simulink library "icc_lib_avg_path1_n1"  (R2018b)
settings: Solver=VariableStepAuto  StartTime=0.0  StopTime=10.0  RelTol=1e-3
undefined symbols (not defined in the file or in its folder): icc_lib_avg_path, path1
libraries: simulink x34, simulink_extras x8, $bdroot x2
(part 4 of 4)

== stateflow chart icc_lib_avg_path1_n1/ICC7_egm/Chart ==
  state block
    en:
    q=4
  state wait
    entry:
    du:
    t2=temporalCount (sec);
  state q0
    en:
    q=0
  state q1
    en:
    q=1
    Sense=1
    exit:
    Sense=0
  state q3
    en:
    q=3
  state q2
    en:
    q=2
  wait -> (junction 82) : [t2>=19.999]{q=0;th=0;vreset=-67.6336;reset}
  (junction 82) -> block [order 2] : [b==1]
  (junction 82) -> q0 [order 1] : [b==0]
  (default) -> wait : {t2=0;}
  q0 -> block [order 3] : [b==1]
  block -> q0 : [b==0]
  q0 -> q1 [order 1] : [v<VT]/{vreset=v; th=0; Vmax=Vm;d2=d2i; reset}
  q0 -> q1 [order 2] : [gv>VF&&v>VT]{ vreset=v; th=v-VT/VF-VT; Vmax=func1(th,Vm);d2=func2(th,d2i);reset}
  q3 -> q0 : [v<VF]{vreset=v; reset}
  q1 -> q2 : [ v >Vmax ]{vreset=v; reset}
  q2 -> q3 : [v<VR]{vreset=v; reset}
  data: vmax function_output double; theta function_input; vm function_input; d2out function_output double; theta function_input; d2in function_input; v input double; q output; vreset output; gv input double; Vmm input; VT input; Vm input; VR input; VF input; th local; Vmax local; t2 local; d2i input; d2 output; b input; Sense output
  events: reset output EITHER_EDGE_EVENT
  function vmax = func1(theta,vm):
    | function vmax = func1(theta,vm)
    | 
    | m=1;
    | 
    | 
    | vmax1=Vm*exp(-m*th);
    | vmax=-25
  function d2out = func2(theta,d2in):
    | function d2out = func2(theta,d2in)
    | 
    | m=1;
    | 
    | 
    | vmax1=Vm*exp(-m*th);
    | %d2out=-0.5
    | d2out=d2in;

== matlab function icc_lib_avg_path1_n1/ICC7_egm/MATLAB Function ==
  data: cfg output
function cfg = fcn()

%d0-o= -0.039651515;
d0= -0.042051515;
d1= 216.5795;
d2= -0.7491129;
d3= -8.890176;
%d3-1= -8.960176;

VT= -67.6;
Vm= -24.3058;
VR= -28.9622;
VF= -66.9799;

cfg=[d0,d1,d2,d3,VT,Vm,VR,VF];

end

== matlab function icc_lib_avg_path1_n1/ICC7_egm/MATLAB Function-freq=22  ==
  data: cfg2 output
function cfg2 = fcn()

%d0-o= -0.039651515;

%d0= -0.042051515;
%d1= 216.5795;
%d2= -0.7491129;
%d3= -8.890176;

%d3-1= -8.960176;

%freq=22
d0=-0.045;
d1=43.5373;
d2=-0.835;
d3=-6.96;


VT= -67.6336;
Vm= -24.1075;
VR= -28.8921;
VF= -66.9586;



cfg2=[d0,d1,d2,d3,VT,Vm,VR,VF];

end

== matlab function icc_lib_avg_path1_n1/ICC7_egm/MATLAB Function-freq=24 ==
  data: cfg2 output
function cfg2 = fcn()

%d0-o= -0.039651515;

%d0= -0.042051515;
%d1= 216.5795;
%d2= -0.7491129;
%d3= -8.890176;

%d3-1= -8.960176;

%freq24
d0=-0.0381;
d1=43.568;
d2=-0.82;
d3=-4.8;


VT= -67.6336;
Vm= -24.1075;
VR= -28.8921;
VF= -66.9586;



cfg2=[d0,d1,d2,d3,VT,Vm,VR,VF];

end

== matlab function icc_lib_avg_path1_n1/ICC7_egm/MATLAB Function-freq=26  ==
  data: cfg2 output
function cfg2 = fcn()

%d0-o= -0.039651515;

%d0= -0.042051515;
%d1= 216.5795;
%d2= -0.7491129;
%d3= -8.890176;

%d3-1= -8.960176;

%freq26
d0=-0.053;
d1=39.5735;
d2=-0.8035;
d3=-4.69678;


VT= -67.6336;
Vm= -24.1075;
VR= -28.8921;
VF= -66.9586;



cfg2=[d0,d1,d2,d3,VT,Vm,VR,VF];

end

== matlab function icc_lib_avg_path1_n1/ICC7_egm/MATLAB Function-freq=26-o  ==
  data: cfg2 output
function cfg2 = fcn()

%d0-o= -0.039651515;

%d0= -0.042051515;
%d1= 216.5795;
%d2= -0.7491129;
%d3= -8.890176;

%d3-1= -8.960176;

%freq26
d0=-0.053;
d1=39.5735;
d2=-0.8035;
d3=-4.69678;


VT= -67.6336;
Vm= -24.1075;
VR= -28.8921;
VF= -66.9586;



cfg2=[d0,d1,d2,d3,VT,Vm,VR,VF];

end

== matlab function icc_lib_avg_path1_n1/ICC7_egm/MATLAB Function1-freq=20  ==
  data: cfg2 output
function cfg2 = fcn()

%d0-o= -0.039651515;

%d0= -0.042051515;
%d1= 216.5795;
%d2= -0.7491129;
%d3= -8.890176;

%d3-1= -8.960176;


d0=-0.075;
d1=43.625;
d2=-0.88;
d3=-8.65;


VT= -67.6336;
Vm= -24.1075;
VR= -28.8921;
VF= -66.9586;



cfg2=[d0,d1,d2,d3,VT,Vm,VR,VF];

end

== stateflow chart icc_lib_avg_path1_n1/ICC6_egm/Chart ==
  state block
    en:
    q=4
  state wait
    entry:
    du:
    t2=temporalCount (sec);
  state q0
    en:
    q=0
  state q1
    en:
    q=1
    Sense=1
    exit:
    Sense=0
  state q3
    en:
    q=3
  state q2
    en:
    q=2
  wait -> (junction 82) : [t2>=19.999]{q=0;th=0;vreset=-67.6336;reset}
  (junction 82) -> block [order 2] : [b==1]
  (junction 82) -> q0 [order 1] : [b==0]
  (default) -> wait : {t2=0;}
  q0 -> block [order 3] : [b==1]
  block -> q0 : [b==0]
  q0 -> q1 [order 1] : [v<VT]/{vreset=v; th=0; Vmax=Vm;d2=d2i; reset}
  q0 -> q1 [order 2] : [gv>VF&&v>VT]{ vreset=v; th=v-VT/VF-VT; Vmax=func1(th,Vm);d2=func2(th,d2i);reset}
  q3 -> q0 : [v<VF]{vreset=v; reset}
  q1 -> q2 : [ v >Vmax ]{vreset=v; reset}
  q2 -> q3 : [v<VR]{vreset=v; reset}
  data: vmax function_output double; theta function_input; vm function_input; d2out function_output double; theta function_input; d2in function_input; v input double; q output; vreset output; gv input double; Vmm input; VT input; Vm input; VR input; VF input; th local; Vmax local; t2 local; d2i input; d2 output; b input; Sense output
  events: reset output EITHER_EDGE_EVENT
  function vmax = func1(theta,vm):
    | function vmax = func1(theta,vm)
    | 
    | m=1;
    | 
    | 
    | vmax1=Vm*exp(-m*th);
    | vmax=-25
  function d2out = func2(theta,d2in):
    | function d2out = func2(theta,d2in)
    | 
    | m=1;
    | 
    | 
    | vmax1=Vm*exp(-m*th);
    | %d2out=-0.5
    | d2out=d2in;

== matlab function icc_lib_avg_path1_n1/ICC6_egm/MATLAB Function ==
  data: cfg output
function cfg = fcn()

%d0-o= -0.039651515;
d0= -0.042051515;
d1= 216.5795;
d2= -0.7491129;
d3= -8.890176;
%d3-1= -8.960176;

VT= -67.6;
Vm= -24.3058;
VR= -28.9622;
VF= -66.9799;

cfg=[d0,d1,d2,d3,VT,Vm,VR,VF];

end

== matlab function icc_lib_avg_path1_n1/ICC6_egm/MATLAB Function-freq=22  ==
  data: cfg2 output
function cfg2 = fcn()

%d0-o= -0.039651515;

%d0= -0.042051515;
%d1= 216.5795;
%d2= -0.7491129;
%d3= -8.890176;

%d3-1= -8.960176;

%freq=22
d0=-0.045;
d1=43.5373;
d2=-0.835;
d3=-6.96;


VT= -67.6336;
Vm= -24.1075;
VR= -28.8921;
VF= -66.9586;



cfg2=[d0,d1,d2,d3,VT,Vm,VR,VF];

end

== matlab function icc_lib_avg_path1_n1/ICC6_egm/MATLAB Function-freq=24 ==
  data: cfg2 output
function cfg2 = fcn()

%d0-o= -0.039651515;

%d0= -0.042051515;
%d1= 216.5795;
%d2= -0.7491129;
%d3= -8.890176;

%d3-1= -8.960176;

%freq24
d0=-0.0381;
d1=43.568;
d2=-0.82;
d3=-4.8;


VT= -67.6336;
Vm= -24.1075;
VR= -28.8921;
VF= -66.9586;



cfg2=[d0,d1,d2,d3,VT,Vm,VR,VF];

end

== matlab function icc_lib_avg_path1_n1/ICC6_egm/MATLAB Function-freq=26  ==
  data: cfg2 output
function cfg2 = fcn()

%d0-o= -0.039651515;

%d0= -0.042051515;
%d1= 216.5795;
%d2= -0.7491129;
%d3= -8.890176;

%d3-1= -8.960176;

%freq26
d0=-0.053;
d1=39.5735;
d2=-0.8035;
d3=-4.69678;


VT= -67.6336;
Vm= -24.1075;
VR= -28.8921;
VF= -66.9586;



cfg2=[d0,d1,d2,d3,VT,Vm,VR,VF];

end

== matlab function icc_lib_avg_path1_n1/ICC6_egm/MATLAB Function-freq=26-o  ==
  data: cfg2 output
function cfg2 = fcn()

%d0-o= -0.039651515;

%d0= -0.042051515;
%d1= 216.5795;
%d2= -0.7491129;
%d3= -8.890176;

%d3-1= -8.960176;

%freq26
d0=-0.053;
d1=39.5735;
d2=-0.8035;
d3=-4.69678;


VT= -67.6336;
Vm= -24.1075;
VR= -28.8921;
VF= -66.9586;



cfg2=[d0,d1,d2,d3,VT,Vm,VR,VF];

end

== matlab function icc_lib_avg_path1_n1/ICC6_egm/MATLAB Function1-freq=20  ==
  data: cfg2 output
function cfg2 = fcn()

%d0-o= -0.039651515;

%d0= -0.042051515;
%d1= 216.5795;
%d2= -0.7491129;
%d3= -8.890176;

%d3-1= -8.960176;


d0=-0.075;
d1=43.625;
d2=-0.88;
d3=-8.65;


VT= -67.6336;
Vm= -24.1075;
VR= -28.8921;
VF= -66.9586;



cfg2=[d0,d1,d2,d3,VT,Vm,VR,VF];

end

== stateflow chart icc_lib_avg_path1_n1/path_EGM1/Path ==
  state Relay_cell1
  state Relay_cell2
  state Wait_cell1
    du:
    t1=temporalCount(sec);
    ex:
    t1=0;
  state Idle
  state Wait_cell2
    du:
    t2=temporalCount(sec);
    ex:
    t2=0;
  state Annihilate
  Relay_cell2 -> Idle : after(0.1, sec) /
      | {relay2 = 0;}
  Wait_cell2 -> Relay_cell2 : [t2>=0.3]{relay2 = 1;
      | last = 2;}
  Relay_cell1 -> Idle : after(0.1, sec) /
      | {relay1 = 0;}
  Wait_cell1 -> Relay_cell1 : [t1>=0.3]{relay1 = 1;
      | last = 1;}
  (default) -> Idle : {t1=0; t2=0;}
  Idle -> Wait_cell1 [order 2] : [mode1 == 1 ...
      | && mode2 ==0 ]
  Idle -> Wait_cell2 [order 3] : [mode2 == 1 ...
      | && mode1 == 0]
  Idle -> Annihilate [order 1] : [mode1 == 2 ...
      | && mode2 == 2]
  Annihilate -> Idle : [mode1 ~= 2 ...
      | && mode2 ~= 2] /
      | {last = 0;}
  data: mode1 input; mdelay1 input; mode2 input; mdelay2 input; relay1 output; relay2 output; last local =0; cell1_mode_delayed local; cell2_mode_delayed local; t1 output; t2 output

== stateflow chart icc_lib_avg_path1_n1/EGM1/Path2 ==
  state EGM1
    state De_wave_i [parallel]
      settings: executionOrder=1
      state Idle
        en:
        egm_i = 0;
      state Active
        du:
        egm_i  = EGM(cvi,xi,yi,xj,yj,t1,8,10,1,C);
      EGM1.De_wave_i.Idle -> EGM1.De_wave_i.Active : [t1~=0]
      (default) -> EGM1.De_wave_i.Idle
      EGM1.De_wave_i.Active -> EGM1.De_wave_i.Idle : [t1==0]
    state De_wave_j [parallel]
      settings: executionOrder=2
      state Idle
        en:
        egm_j = 0;
      state Active
        du:
        egm_j = EGM(cvj,xj,yj,xi,yi,t2,8,10,1,C);
      EGM1.De_wave_j.Idle -> EGM1.De_wave_j.Active : [t2~=0]
      (default) -> EGM1.De_wave_j.Idle
      EGM1.De_wave_j.Active -> EGM1.De_wave_j.Idle : [t2==0]
  (default) -> EGM1
  data: cv1in function_input; x1in function_input; y1in function_input; x2in function_input; y2in function_input; t1in function_input; xe function_input; ye function_input; ze function_input; Cin function_input; Potential_d function_output; xi input; yi input; xj input; yj input; cvi input; cvj input; t1 input; t2 input; C input; egm_i output; egm_j output
  function Potential_d = EGM(cv1in,x1in,y1in,x2in,y2in,t1in,xe,ye,ze,Cin):
    | function Potential_d = EGM(cv1in,x1in,y1in,x2in,y2in,t1in,xe,ye,ze,Cin)
    |     %#codegen
    |     % % The distance (mm) between the electrodes and the activation in z
    |     % direction
    |     % Compute theta2: the angle between (x1,y1)-->(x2,y2) and x axis;
    |     cos_theta2=(x2in-x1in)/sqrt((x2in-x1in)^2+(y2in-y1in)^2);
    |     sin_theta2=(y1in-y2in)/sqrt((x2in-x1in)^2+(y2in-y1in)^2);
    |     if cos_theta2~=0
    |     tan_theta2=(y1in-y2in)/(x2in-x1in);
    |     else
    |      tan_theta2=0;   
    |     end
    |     
    | %     N=length(electrodein)-4; % The number of (x,y,z) of total micro electrodes;
    | %     
    | %     vtip=electrodein(length(electrodein)); % The number of micro electrodes of the ventricular tip part;
    | %     vring=electrodein(length(electrodein)-1); % The number of micro electrodes of the ventricular ring part;
    | %     atip=electrodein(length(electrodein)-2); % The number of micro electrodes of the atrial tip part;
    | %     aring=electrodein(length(electrodein)-3); % The number of micro electrodes of the atrial ring part;
    | %     Potential_d=zeros(1,4); % To store the EGM sensed by atrial ring, tip, ventricular ring and tip part;
    | %     p=zeros(1,N/3); % To store the signals sensed by all the micro electrodes;
    | 
    |     L=1; % weighting factor of the longitudinal dipole
    |     T=0.1; % weighting factor of the transversal dipole
    |     % Only when the path is active, can the cells contribute to the EGM
    | %     m=0;
    | %     for j=1:3:(N-2)
    |     % The location of the micro electrode
    | %     x3=electrodein(j);
    | %     y3=electrodein(j+1);
    | %     zin=electrodein(j+2);
    |     % The closest point to the micro electrode
    |     if cos_theta2~=0
    |         y4=(y2in+tan_theta2*(x2in-xe+tan_theta2*ye))/(1+tan_theta2^2);
    |         x4=tan_theta2*y4-tan_theta2*ye+xe;
    |     else
    |         y4=ye;
    |         x4=x1in;
    |     end
    |     d=sqrt((xe-x4)^2+(ye-y4)^2+ze^2);
    | 
    |     x11=x1in+cv1in*t1in*cos_theta2; % the dipole position
    |     y11=y1in-cv1in*t1in*sin_theta2;
    |     % Compute theta1: the angle between (x11,y11)-->(x3,y3) and x axis;
    |     if xe==x11 && ye==y11
    |      cos_theta1=0;
    |      sin_theta1=0;
    |     else
    |         cos_theta1=(xe-x11)/sqrt((xe-x11)^2+(ye-y11)^2);
    |         sin_theta1=(ye-y11)/sqrt((xe-x11)^2+(ye-y11)^2);
    |     end
    |     % alfa=theta1+theta2, the angle between (x11,y11)-->(x3,y3) and (x11,y11)-->(x2,y2)
    |     cos_alfa = cos_theta1*cos_theta2 - sin_theta1*sin_theta2;
    | 
    |     h1=sqrt((x4-x11)^2+(y4-y11)^2)*sign(cos_alfa); % the distance between the dipole and (x4,y4), when the dipole is approaching, h1>0;
    |     r1=sqrt((d^2+h1^2)); % the distance between the dipole and the micro electrode;
    |     EGML1=L*h1/(r1^3);
    |     EGMT1=(-1)*T*d/(r1^3);
    |     EGMall=EGML1+EGMT1;
    | %     m=m+1;
    | %     p(m) =EGMall*Cin;
    |     Potential_d=EGMall*Cin;
    | %     end
    | %     s=1;
    | %     e=aring;
    | %     Potential_d(1)=sum(p(s:e));
    | %     s=e+1;
    | %     e=s+atip-1;
    | %     Potential_d(2)=sum(p(s:e));
    | %     s=e+1;
    | %     e=s+vring-1;
    | %     Potential_d(3)=sum(p(s:e));
    | %     s=e+1;
    | %     e=s+vtip-1;
    | %     Potential_d(4)=sum(p(s:e));
    | 
    | end

== stateflow chart icc_lib_avg_path1_n1/ICC1_egm_b/Chart ==
  state wait
    entry:
    du:
    t2=temporalCount (sec);
  state q0
    en:
    q=0
  state q1
    en:
    q=1
    Sense=1;
    exit:
    Sense=0;
  state q3
    en:
    q=3
  state q2
    en:
    q=2
  (default) -> wait : {t2=0;}
  wait -> q0 : [t2>=19.999]{q=0;vreset=-67.6336;reset}
  q0 -> q1 [order 1] : [v<VT]/{vreset=v;Vmax=Vm;d2=d2i;reset}
  q0 -> q1 [order 2] : [gv>VF&&v>VT]{ vreset=v; Vmax=Vm;d2=d2i;reset}
  q3 -> q0 : [v<VF]{vreset=v; reset}
  q1 -> q2 : [ v >Vmax ]{vreset=v; reset}
  q2 -> q3 : [v<VR]{vreset=v; reset}
  data: v input double; q output; vreset output; gv input double; VT input; Vm input; VR input; VF input; Vmax local; t2 local; d2i input; d2 output; Sense output
  events: reset output EITHER_EDGE_EVENT

== matlab function icc_lib_avg_path1_n1/ICC1_egm_b/MATLAB Function ==
  data: cfg output
function cfg = fcn()

%d0-o= -0.039651515;
d0= -0.042051515;
d1= 216.5795;
d2= -0.7491129;
d3= -8.890176;
%d3-1= -8.960176;

VT= -67.6;
Vm= -24.3058;
VR= -28.9622;
VF= -66.9799;

cfg=[d0,d1,d2,d3,VT,Vm,VR,VF];

end

== matlab function icc_lib_avg_path1_n1/ICC1_egm_b/MATLAB Function-freq=22  ==
  data: cfg2 output
function cfg2 = fcn()

%d0-o= -0.039651515;

%d0= -0.042051515;
%d1= 216.5795;
%d2= -0.7491129;
%d3= -8.890176;

%d3-1= -8.960176;

%freq=22
d0=-0.045;
d1=43.5373;
d2=-0.835;
d3=-6.96;


VT= -67.6336;
Vm= -24.1075;
VR= -28.8921;
VF= -66.9586;



cfg2=[d0,d1,d2,d3,VT,Vm,VR,VF];

end

== matlab function icc_lib_avg_path1_n1/ICC1_egm_b/MATLAB Function-freq=24 ==
  data: cfg2 output
function cfg2 = fcn()

%d0-o= -0.039651515;

%d0= -0.042051515;
%d1= 216.5795;
%d2= -0.7491129;
%d3= -8.890176;

%d3-1= -8.960176;

%freq24
d0=-0.0381;
d1=43.568;
d2=-0.82;
d3=-4.8;


VT= -67.6336;
Vm= -24.1075;
VR= -28.8921;
VF= -66.9586;



cfg2=[d0,d1,d2,d3,VT,Vm,VR,VF];

end

== matlab function icc_lib_avg_path1_n1/ICC1_egm_b/MATLAB Function-freq=26  ==
  data: cfg2 output
function cfg2 = fcn()

%d0-o= -0.039651515;

%d0= -0.042051515;
%d1= 216.5795;
%d2= -0.7491129;
%d3= -8.890176;

%d3-1= -8.960176;

%freq26
d0=-0.053;
d1=39.5735;
d2=-0.8035;
d3=-4.69678;


VT= -67.6336;
Vm= -24.1075;
VR= -28.8921;
VF= -66.9586;



cfg2=[d0,d1,d2,d3,VT,Vm,VR,VF];

end

== matlab function icc_lib_avg_path1_n1/ICC1_egm_b/MATLAB Function-freq=26-o  ==
  data: cfg2 output
function cfg2 = fcn()

%d0-o= -0.039651515;

%d0= -0.042051515;
%d1= 216.5795;
%d2= -0.7491129;
%d3= -8.890176;

%d3-1= -8.960176;

%freq26
d0=-0.053;
d1=39.5735;
d2=-0.8035;
d3=-4.69678;


VT= -67.6336;
Vm= -24.1075;
VR= -28.8921;
VF= -66.9586;



cfg2=[d0,d1,d2,d3,VT,Vm,VR,VF];

end

== matlab function icc_lib_avg_path1_n1/ICC1_egm_b/MATLAB Function1-freq=20  ==
  data: cfg2 output
function cfg2 = fcn()

%d0-o= -0.039651515;

%d0= -0.042051515;
%d1= 216.5795;
%d2= -0.7491129;
%d3= -8.890176;

%d3-1= -8.960176;


d0=-0.075;
d1=43.625;
d2=-0.88;
d3=-8.65;


VT= -67.6336;
Vm= -24.1075;
VR= -28.8921;
VF= -66.9586;



cfg2=[d0,d1,d2,d3,VT,Vm,VR,VF];

end

== matlab function icc_lib_avg_path1_n1/egm_pace ==
  settings: updateMethod=DISCRETE
  data: time input; pace output; egm_sum input; count input; count output; basetime input; basetime output; c input; c output
function [pace,count,basetime,c] = fcn(time,egm_sum,count,basetime,c)

% persistent count;
% count = 0;
% c = 0;
% basetime = 0;
pace = 0;
if time > 39
    if count == 0
        if abs(egm_sum) > 4.3
            disp("first time------------------------------------");
            disp(time);
            disp(egm_sum);
            count = count + 1;
            basetime = round(time*10)/10;
            disp(count);
            disp(basetime);
%             c=1;
        end

    else
%         disp("second")
        td = round(time*10)/10-basetime;
        if td> 5 & td <= 20 
%             if egm_sum == 0
%                 c = 0;
%             end

%             disp('c value')
%             disp(round(time*10)/10);
%             disp(c)
            if abs(egm_sum) > 4.3            
                if c == 0
                    basetime = round(time*10)/10;
                    disp("second ------------------------------");
                    disp(basetime)
%                     c=1;
                end
            end
        elseif td > 20
            if abs(egm_sum) > 4.3
                disp("update -----------------------------")
                disp(round(time*10)/10);
                basetime = round(time*10)/10;
                pace =0;
            
            else
                disp("pace -------------------------------")
                disp(round(time*10)/10);
                pace = 2;
            end
        end
    end
end


%x = get_param('ICCNetwork9_2_nf_EGM3','SimulationTime');

% function pace = fcn(egm_sum)
%  
% 
% % autoegmh1 = [egm1_2.Time, egm1_2.Data, egm2_3.Data, egm3_6.Data ,egm4_5.Data, egm5_6.Data, egm6_9.Data, egm7_8.Data, egm8_9.Data, egm8_9.Data];
% % autoegmc1 = [egm_c1.Time, egm_c1.Data, egm_c2.Data, egm_c3.Data ,egm_c4.Data, egm_c5.Data, egm_c6.Data, egm_c7.Data, egm_c8.Data, egm_c9.Data];
% autosum = [egm_sum.Time, egm_sum.Data];
% 
% 
% %---------- For EGM SUM detect abnormal delay ----------
% autosum(1:38000,:) = [];
% TbEGM = 40;
% countES = 0;
% P = 0;
% startT = 0;
% endT = 0;
% 
% %---------- EGM SUM Detect abnormal delay ----------
% for i = 1:10000   
%     for j = 2
%         
%         if countES == 0
%             if autosum(i,j) == 0
%                if autosum(i+1,j) ~= 0
% 
%                    startT = round((autosum(i+1,1) - TbEGM),1)
%                    countES = countES+1;
%                    
%                    if startT ~= 0
%                        P = 2;
%                    end
%                    
%                end
%                
%            
%            end 
%         end
%        
%     end
% end
% 
% if egm_sum ~= 0
    
% pace = 1;
% 
% 
% 
% 
% 
% 
% 
% 
% 
% 
% 
% 
%

== matlab function icc_lib_avg_path1_n1/egm_pace1 ==
  settings: updateMethod=DISCRETE
  data: time input; pace output; egm_sum input; count input; count output; basetime input; basetime output
function [pace,count,basetime] = fcn(time,egm_sum,count,basetime)

pace = 0;
if time > 39
    if count == 0
        
        if abs(egm_sum) > 4.3
            disp("first time------------------------------------");
            disp(time);
            disp(egm_sum);
            count = count + 1;
            basetime = round(time*10)/10;
            disp(count);
            disp(basetime);
        end

    else
        
        td = round(time*10)/10-basetime;
        if td> 5 && td <= 20
            
            if abs(egm_sum) > 4.3            
                basetime = round(time*10)/10;
                disp("second ------------------------------");
                disp(basetime)
            end
            
        elseif td > 20
            
            if abs(egm_sum) > 4.3
                disp("update -----------------------------")
                disp(round(time*10)/10);
                basetime = round(time*10)/10;
                pace =0;
            else
                disp("pace -------------------------------")
                disp(round(time*10)/10);
                pace = 2;
            end
            
        end
        
    end
end
